simulink model "Sim_Double_P2Q_FM_N_dis_zero"  (R2017a)
settings: Solver=ode3  StartTime=0.0  StopTime=10  FixedStep=0.01  RelTol=1e-3  EnableMultiTasking=on
libraries: aerolibanimutils x1
settings Model: Creator=GeoLee  LastModifiedBy=gmh_n
settings DataIOCC: SaveFormat=Array  SaveOutput=off  SaveTime=off
settings OptimizationCC: LifeSpan=inf
settings DebuggingCC: SFUnexpectedBacktrackingDiag=warning  SFNoUnconditionalDefaultTransitionDiag=warning  SFExecutionAtInitializationDiag=none
settings HardwareCC: ProdBitPerPointer=32  ProdBitPerSizeT=32  ProdBitPerPtrDiffT=32  ProdLargestAtomicFloat=None  ProdIntDivRoundTo=Undefined  ProdEndianess=Unspecified  ProdWordSize=32  ProdHWDeviceType=32-bit Generic
settings ModelReferenceCC: PropagateSignalLabelsOutOfModel=off
settings GRTTargetCC: TargetLangStandard=C89/C90 (ANSI)  GeneratePreprocessorConditionals=Disable all
settings ConfigComp: CovMetricSettings=dw  CovHtmlReporting=on  CovSaveCumulativeToWorkspaceVar=on  CovSaveSingleToWorkspaceVar=on  CovExternalEMLEnable=off

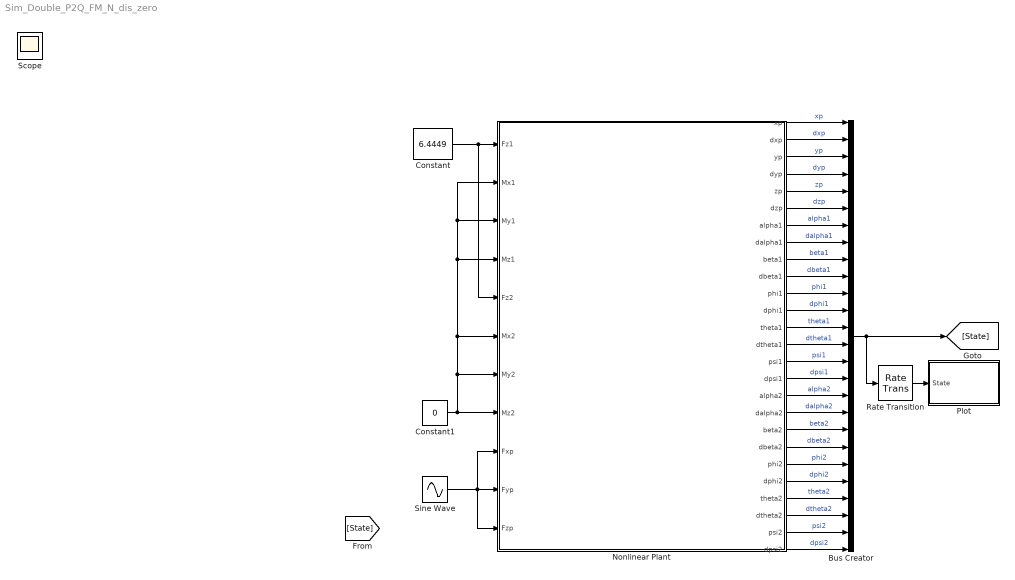
== system Sim_Double_P2Q_FM_N_dis_zero ==
  Bus Creator : BusCreator  Inputs=26
  Constant : Constant  Value=6.4449
  Constant1 : Constant  Value=0
  Nonlinear Plant : Subsystem  mask{xp0=0, yp0=0, zp0=0, a10=0, b10=45, a20=180, b20=45}
      mask prompts: xp0 "initial position of load xp0"; yp0 "initial position of load yp0"; zp0 "initial position of load zp0"; a10 "alpha10(deg) (default: 0) (0~360)"; b10 "beta10(deg) (default: 45) (cannot be 0)"; a20 "alpha20(deg) (default: 180) (0~360)"; b20 "beta10(deg) (default: 45) (cannot be 0)"
      mask Display:
      | image('quads_double.png')
      | port_label('input', 1, 'Fz1')
      | port_label('input', 2, 'Mx1')
      | port_label('input', 3, 'My1')
      | port_label('input', 4, 'Mz1')
      | port_label('input', 5, 'Fz2')
      | port_label('input', 6, 'Mx2')
      | port_label('input', 7, 'My2')
      | port_label('input', 8, 'Mz2')
      | port_label('input', 9, 'Fxp')
      | port_label('input', 10, 'Fyp')
      | port_label('input', 11, 'Fzp')
      | port_label('output', 1, 'xp')
      | port_label('output', 2, 'dxp')
      | port_label('output', 3, 'yp')
      | port_label('output', 4, 'dyp')
      | port_label('output', 5, 'zp')
      | port_label('output', 6, 'dzp')
      | port_label('output', 7, 'alpha1')
      | port_label('output', 8, 'dalpha1')
      | port_label('output', 9, 'beta1')
      | port_label('output', 10, 'dbeta1')
      | port_label('output', 11, 'phi1')
      | port_label('output', 12, 'dphi1')
      | port_label('output', 13, 'theta1')
      | port_label('output', 14, 'dtheta1')
      | port_label('output', 15, 'psi1')
      | port_label('output', 16, 'dpsi1')
      | port_label('output', 17, 'alpha2')
      | port_label('output', 18, 'dalpha2')
      | port_label('output', 19, 'beta2')
      | port_label('output', 20, 'dbeta2')
      | port_label('output', 21, 'phi2')
      | port_label('output', 22, 'dphi2')
      | port_label('output', 23, 'theta2')
      | port_label('output', 24, 'dtheta2')
      | port_label('output', 25, 'psi2')
      | port_label('output', 26, 'dpsi2')
  Plot : Stateflow chart  TreatAsAtomicUnit=on
  Rate Transition : RateTransition  OutPortSampleTime=0.05
  Sine Wave : Sin  Amplitude=0.5  Frequency=2*pi*1  SampleTime=0
  Scope : Scope
  wires:
  Nonlinear Plant/1(xp) -> Bus Creator/1  "xp"
  Nonlinear Plant/2(dxp) -> Bus Creator/2  "dxp"
  Nonlinear Plant/3(yp) -> Bus Creator/3  "yp"
  Nonlinear Plant/4(dyp) -> Bus Creator/4  "dyp"
  Nonlinear Plant/5(zp) -> Bus Creator/5  "zp"
  Nonlinear Plant/6(dzp) -> Bus Creator/6  "dzp"
  Nonlinear Plant/7(alpha1) -> Bus Creator/7  "alpha1"
  Nonlinear Plant/8(dalpha1) -> Bus Creator/8  "dalpha1"
  Nonlinear Plant/9(beta1) -> Bus Creator/9  "beta1"
  Nonlinear Plant/10(dbeta1) -> Bus Creator/10  "dbeta1"
  Nonlinear Plant/11(phi1) -> Bus Creator/11  "phi1"
  Nonlinear Plant/12(dphi1) -> Bus Creator/12  "dphi1"
  Nonlinear Plant/13(theta1) -> Bus Creator/13  "theta1"
  Nonlinear Plant/14(dtheta1) -> Bus Creator/14  "dtheta1"
  Nonlinear Plant/15(psi1) -> Bus Creator/15  "psi1"
  Nonlinear Plant/16(dpsi1) -> Bus Creator/16  "dpsi1"
  Nonlinear Plant/17(alpha2) -> Bus Creator/17  "alpha2"
  Nonlinear Plant/18(dalpha2) -> Bus Creator/18  "dalpha2"
  Nonlinear Plant/19(beta2) -> Bus Creator/19  "beta2"
  Nonlinear Plant/20(dbeta2) -> Bus Creator/20  "dbeta2"
  Nonlinear Plant/21(phi2) -> Bus Creator/21  "phi2"
  Nonlinear Plant/22(dphi2) -> Bus Creator/22  "dphi2"
  Nonlinear Plant/23(theta2) -> Bus Creator/23  "theta2"
  Nonlinear Plant/24(dtheta2) -> Bus Creator/24  "dtheta2"
  Nonlinear Plant/25(psi2) -> Bus Creator/25  "psi2"
  Nonlinear Plant/26(dpsi2) -> Bus Creator/26  "dpsi2"
  Bus Creator/1 -> Rate Transition/1, [State]
  Rate Transition/1 -> Plot/1(State)
  Constant/1 -> Nonlinear Plant/5(Fz2), Nonlinear Plant/1(Fz1)
  Sine Wave/1 -> Nonlinear Plant/9(Fxp), Nonlinear Plant/11(Fzp), Nonlinear Plant/10(Fyp)
  Constant1/1 -> Nonlinear Plant/7(My2), Nonlinear Plant/6(Mx2), Nonlinear Plant/4(Mz1), Nonlinear Plant/3(My1), Nonlinear Plant/2(Mx1), Nonlinear Plant/8(Mz2)

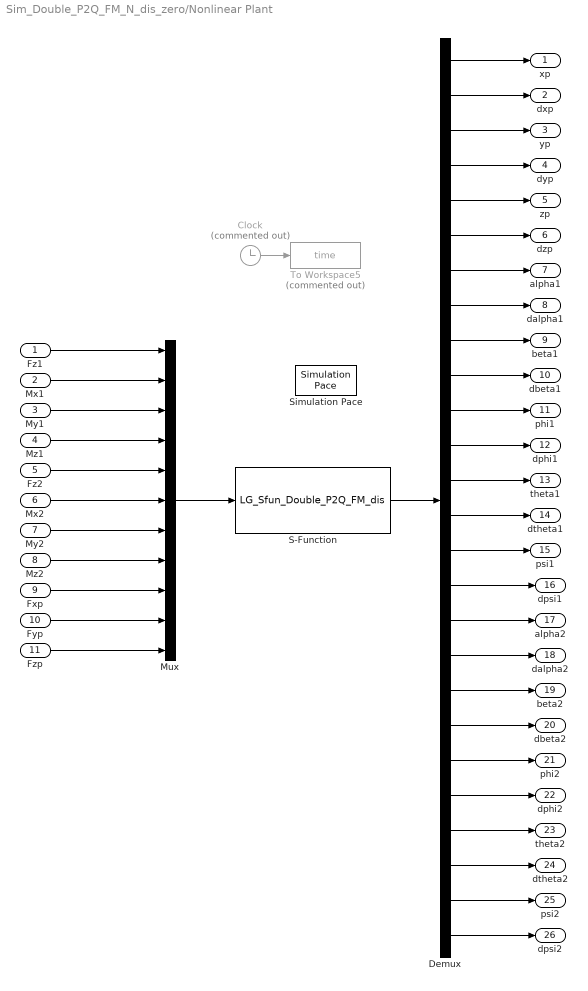
== system Sim_Double_P2Q_FM_N_dis_zero/Nonlinear Plant ==
  Fz1 : Inport
  Mx1 : Inport  Port=2
  My1 : Inport  Port=3
  Mz1 : Inport  Port=4
  Fz2 : Inport  Port=5
  Mx2 : Inport  Port=6
  My2 : Inport  Port=7
  Mz2 : Inport  Port=8
  Fxp : Inport  Port=9
  Fyp : Inport  Port=10
  Fzp : Inport  Port=11
  Clock : Clock  Commented=on
  Demux : Demux  Outputs=26
  Mux : Mux  Inputs=11
  S-Function : S-Function  FunctionName=LG_Sfun_Double_P2Q_FM_dis  Parameters=xp0,yp0,zp0,a10,b10,a20,b20  SFunctionDeploymentMode=off  EnableBusSupport=off
  Simulation Pace : aerolibanimutils/Simulation Pace  SimulationPace=1  SleepMode=MATLAB Thread  OutputPaceError=off  SampleTime=-1
  To Workspace5 : ToWorkspace  Commented=on  VariableName=time  SampleTime=-1
  xp : Outport
  dxp : Outport  Port=2
  yp : Outport  Port=3
  dyp : Outport  Port=4
  zp : Outport  Port=5
  dzp : Outport  Port=6
  alpha1 : Outport  Port=7
  dalpha1 : Outport  Port=8
  beta1 : Outport  Port=9
  dbeta1 : Outport  Port=10
  phi1 : Outport  Port=11
  dphi1 : Outport  Port=12
  theta1 : Outport  Port=13
  dtheta1 : Outport  Port=14
  psi1 : Outport  Port=15
  dpsi1 : Outport  Port=16
  alpha2 : Outport  Port=17
  dalpha2 : Outport  Port=18
  beta2 : Outport  Port=19
  dbeta2 : Outport  Port=20
  phi2 : Outport  Port=21
  dphi2 : Outport  Port=22
  theta2 : Outport  Port=23
  dtheta2 : Outport  Port=24
  psi2 : Outport  Port=25
  dpsi2 : Outport  Port=26
  wires:
  Demux/10 -> dbeta1/1
  My2/1 -> Mux/7
  Demux/24 -> dtheta2/1
  Demux/23 -> theta2/1
  Demux/22 -> dphi2/1
  Demux/21 -> phi2/1
  Demux/20 -> dbeta2/1
  Demux/19 -> beta2/1
  Demux/18 -> dalpha2/1
  Mz1/1 -> Mux/4
  Demux/16 -> dpsi1/1
  Demux/14 -> dtheta1/1
  Demux/15 -> psi1/1
  Mx2/1 -> Mux/6
  Demux/17 -> alpha2/1
  Demux/13 -> theta1/1
  Demux/12 -> dphi1/1
  Demux/8 -> dalpha1/1
  Demux/5 -> zp/1
  My1/1 -> Mux/3
  Demux/9 -> beta1/1
  Demux/6 -> dzp/1
  Demux/11 -> phi1/1
  Demux/25 -> psi2/1
  Demux/7 -> alpha1/1
  Demux/4 -> dyp/1
  Demux/3 -> yp/1
  Mx1/1 -> Mux/2
  Demux/1 -> xp/1
  Demux/2 -> dxp/1
  Demux/26 -> dpsi2/1
  Mz2/1 -> Mux/8
  S-Function/1 -> Demux/1
  Mux/1 -> S-Function/1
  Fz1/1 -> Mux/1
  Fz2/1 -> Mux/5
  Clock/1 -> To Workspace5/1
  Fxp/1 -> Mux/9
  Fyp/1 -> Mux/10
  Fzp/1 -> Mux/11

== stateflow chart Sim_Double_P2Q_FM_N_dis_zero/Plot ==
  state Plot
    entry:
    fig = ml.figure();
    phandles = ml.LG_plot_initial( fig,State);
    du:
    ml.LG_plot_update(fig,State,phandles);
  (default) -> Plot
  data: State input double size=26; fig local ml; phandles local ml
